simulink model "ayazLiftingBody_th"  (R2018b)
settings: Solver=VariableStepAuto  StartTime=0.0  StopTime=10.0  RelTol=1e-3
values from neighbouring files (symbols this model uses):
  elevonCmds = [0 0]    [ayazLiftingBody_ts.m]
  flow = [1 0 0]    [ayazLiftingBody_ts.m]
  ten1Vec = [0 0 -1]    [ayazLiftingBody_ts.m]
  ten2Vec = [0 0 -1]    [ayazLiftingBody_ts.m]
  ten3Vec = [0 0 -1]    [ayazLiftingBody_ts.m]
libraries: ayazLiftingBody_cl x1
settings Model: Creator=mcobb  LastModifiedBy=mcobb

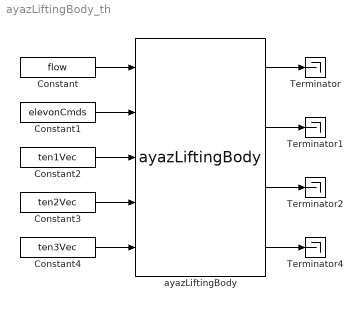
== system ayazLiftingBody_th ==
  Constant : Constant  Value=flow
  Constant1 : Constant  Value=elevonCmds
  Constant2 : Constant  Value=ten1Vec
  Constant3 : Constant  Value=ten2Vec
  Constant4 : Constant  Value=ten3Vec
  Terminator{,1..2,4} (4 alike) : Terminator
  ayazLiftingBody : ayazLiftingBody_cl/ayazLiftingBody  SystemSampleTime=-1
  wires:
  Constant/1 -> ayazLiftingBody/1
  Constant1/1 -> ayazLiftingBody/2
  Constant2/1 -> ayazLiftingBody/3
  Constant3/1 -> ayazLiftingBody/4
  Constant4/1 -> ayazLiftingBody/5
  ayazLiftingBody/1 -> Terminator/1
  ayazLiftingBody/2 -> Terminator1/1
  ayazLiftingBody/3 -> Terminator2/1
  ayazLiftingBody/4 -> Terminator4/1
